simulink model "Mechanical_model_of_servo"  (R2013b)
settings: Solver=ode45  StartTime=0.0  StopTime=1  RelTol=1e-3
values from neighbouring files (symbols this model uses):
  B = 0.1e-3    (= 0.0001)    [Mechanical_model_of_servo_Variables.m]
  J = 0.1    [Mechanical_model_of_servo_Variables.m]
  Tf = 0.1    [Mechanical_model_of_servo_Variables.m]
libraries: powerlib x1
settings Model: Creator=User  LastModifiedBy=User

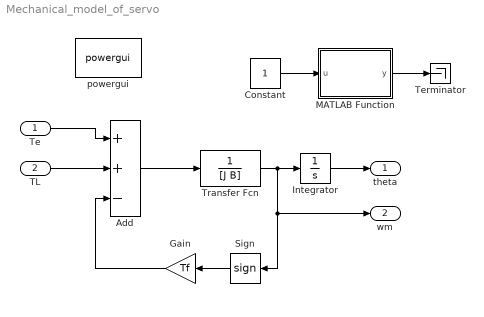
== system Mechanical_model_of_servo ==
  Te : Inport
  TL : Inport  Port=2
  Add : Sum  Inputs=++-
  Constant : Constant
  Gain : Gain  Gain=Tf
  Integrator : Integrator
  MATLAB Function : MATLAB Function  TreatAsAtomicUnit=on
  Sign : Signum
  Terminator : Terminator
  Transfer Fcn : TransferFcn  Denominator=[J B]
  powergui : powerlib/powergui  Priority=1  SimulationMode=Continuous  SolverType=Tustin  SampleTime=50e-6  frequency=60  SPID=off  DisableSnubberDevices=off  DisableRonSwitches=off  DisableVfSwitches=off  SwTol=0  Interpol=off  DisplayEquations=off  frequencyindice=60  Pbase=100e6  ErrMax=1e-4  Iterations=50  UnitsV=kV  UnitsW=MW  FunctionMessages=off  echomessages=off  HookPort=off  EnableUseOfTLC=off  x0status=blocks  RestoreLinks=warning  ResistiveCurrentMeasurement=off  Frange=[0:2:500]  Ylog=off  Xlog=on  ShowGrid=off  save=off  variable=ZData  ZoomFFT=off  StartTime=0.0  cycles=1  DisplayStyle=1  fundamental=60  FreqAxis=off  MaxFrequency=1000  frequencyindicesteady=1  RmsSteady=1  display=off  Ts=0  methode=off
  theta : Outport
  wm : Outport  Port=2
  wires:
  Te/1 -> Add/1
  TL/1 -> Add/2
  Constant/1 -> MATLAB Function/1(u)
  MATLAB Function/1(y) -> Terminator/1
  Add/1 -> Transfer Fcn/1
  Transfer Fcn/1 -> wm/1, Sign/1, Integrator/1
  Integrator/1 -> theta/1
  Sign/1 -> Gain/1
  Gain/1 -> Add/3

== matlab function Mechanical_model_of_servo/MATLAB Function ==
  data: u input; y output
function y = fcn(u)
u=0;
y=0;
J=0.1; %kg/m^3
B=0.1e-3; %Nm.s/rad
Tf=0.1; %static friction
%#codegen

y = u;
